simulink model "rtdemo1_init"  (Simulink 7.7)
settings: Solver=ode4  StartTime=0.0  StopTime=inf  FixedStep=0.001  RelTol=1e-3
libraries: opal_lib x2, simulink x1
Description:
  | Model of a simple control system for use iin training.
settings Model: Creator=Paul Baracos  LastModifiedBy=DanielOBrien
settings DataIOCC: LimitDataPoints=off  SaveOutput=off  SaveTime=off  SignalLoggingName=sigsOut
settings OptimizationCC: BlockReduction=off  BooleanDataType=off  InitFltsAndDblsToZero=on
settings DebuggingCC: SaveWithParameterizedLinksMsg=none  SignalResolutionControl=TryResolveAllWithWarning  SolverPrmCheckMsg=none  MultiTaskDSMMsg=warning  MultiTaskCondExecSysMsg=none  StrictBusMsg=None
settings HardwareCC: TargetUnknown=on
settings CodeAppCC: CustomSymbolStrType=$N$R$M_T
settings GRTTargetCC: TargetFcnLib=ansi_tfl_tmw.mat  TargetFunctionLibrary=C89/C90 (ANSI)

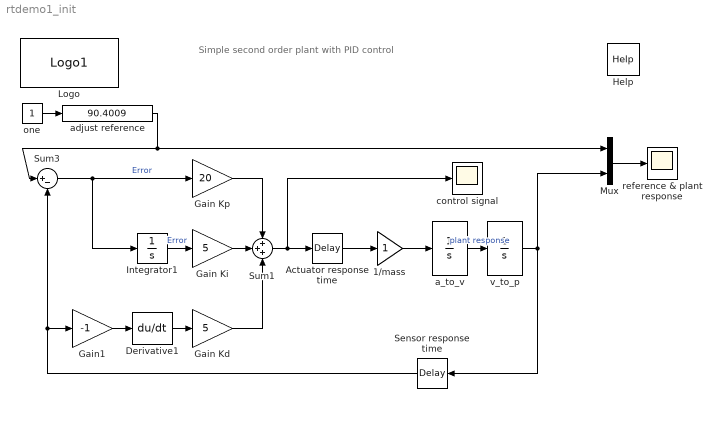
== system rtdemo1_init ==
  note: Simple second order plant with PID control
  1/mass : Gain  SaturateOnIntegerOverflow=on  OutDataTypeStr=Inherit: Same as input  ParamDataTypeStr=Inherit: Same as input
  Actuator response time : TransportDelay  DelayTime=0.005  BufferSize=1+ceil(0.005/eval(get_param(bdroot, 'FixedStep')))
  Derivative1 : Derivative
  Gain Kd : Gain  Gain=5  SaturateOnIntegerOverflow=on  OutDataTypeStr=Inherit: Same as input  ParamDataTypeStr=Inherit: Same as input
  Gain Ki : Gain  Gain=5  SaturateOnIntegerOverflow=on  OutDataTypeStr=Inherit: Same as input  ParamDataTypeStr=Inherit: Same as input
  Gain Kp : Gain  Gain=20  SaturateOnIntegerOverflow=on  OutDataTypeStr=Inherit: Same as input  ParamDataTypeStr=Inherit: Same as input
  Gain1 : Gain  Gain=-1  SaturateOnIntegerOverflow=on  OutDataTypeStr=Inherit: Same as input  ParamDataTypeStr=Inherit: Same as input
  Help : opal_lib/Help  docfile=Examples/Basic/rtdemo1/rtdemo1.htm
  Integrator1 : Integrator
  Logo : opal_lib/Logo1  vide=[]
  Mux : Mux  Inputs=2
  Sensor response time : TransportDelay  DelayTime=0.005  BufferSize=1+ceil(0.005/eval(get_param(bdroot, 'FixedStep')))
  Sum1 : Sum  Inputs=+++  SaturateOnIntegerOverflow=on  InputSameDT=on  OutDataTypeStr=Inherit: Same as first input
  Sum3 : Sum  Inputs=|+-  SaturateOnIntegerOverflow=on  InputSameDT=on  OutDataTypeStr=Inherit: Same as first input
  a_to_v : Integrator
  adjust reference : simulink/Math Operations/Slider Gain  low=0  gain=90.4009  high=100
  control signal : Scope
      settings: YMin=-200  YMax=200  SaveName=controlSignal
  one : Constant
  reference & plant response : Scope
      settings: Tag=op_tm_save_it  TimeRange=10  YMin=0  YMax=160  SaveName=referenceAndPlant
  v_to_p : Integrator  LimitOutput=on  UpperSaturationLimit=200  LowerSaturationLimit=0
  wires:
  v_to_p/1 -> Sensor response time/1, Mux/2
  Sum3/1 -> Integrator1/1, Gain Kp/1  "Error"
  Gain Kp/1 -> Sum1/1
  Integrator1/1 -> Gain Ki/1  "Error"
  Derivative1/1 -> Gain Kd/1
  Gain Ki/1 -> Sum1/2
  Gain1/1 -> Derivative1/1
  Gain Kd/1 -> Sum1/3
  Sum1/1 -> Actuator response time/1, control signal/1
  Actuator response time/1 -> 1/mass/1
  a_to_v/1 -> v_to_p/1  "plant response"
  1/mass/1 -> a_to_v/1
  Mux/1 -> reference & plant response/1
  adjust reference/1 -> Mux/1, Sum3/1
  one/1 -> adjust reference/1
  Sensor response time/1 -> Gain1/1, Sum3/2
